simulink model "Flatten2_export"  (Simulink 7.9)
settings: Solver=FixedStepDiscrete  StartTime=0.0  StopTime=100000000.0  FixedStep=1  RelTol=1e-3
settings Model: Creator=boakes  LastModifiedBy=boakes
settings OptimizationCC: InlineParams=on  InlineInvariantSignals=on  EnhancedBackFolding=on

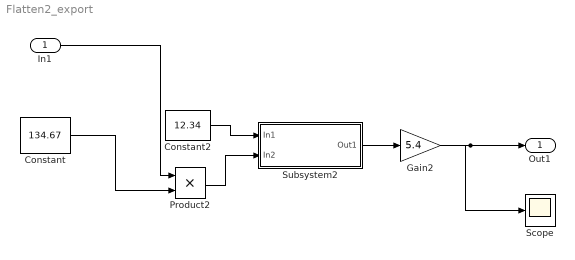
== system Flatten2_export ==
  In1 : Inport
  Constant : Constant  Value=134.67
  Constant2 : Constant  Value=12.34
  Gain2 : Gain  Gain=5.4
  Product2 : Product  RndMeth=Zero
  Scope : Scope
      settings: SaveName=ScopeData2
  Subsystem2 : Subsystem
  Out1 : Outport
  wires:
  Constant/1 -> Product2/2
  Constant2/1 -> Subsystem2/1(In1)
  In1/1 -> Product2/1
  Gain2/1 -> Out1/1, Scope/1
  Product2/1 -> Subsystem2/2(In2)
  Subsystem2/1(Out1) -> Gain2/1

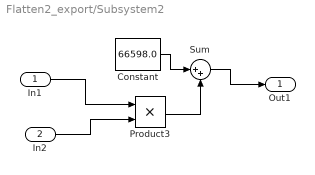
== system Flatten2_export/Subsystem2 ==
  In1 : Inport
  In2 : Inport  Port=2
  Constant : Constant  Value=66598.0
  Product3 : Product  RndMeth=Zero
  Sum : Sum  Inputs=|++
  Out1 : Outport
  wires:
  Constant/1 -> Sum/1
  Product3/1 -> Sum/2
  Sum/1 -> Out1/1
  In2/1 -> Product3/2
  In1/1 -> Product3/1
